simulink model "x_33_sim"  (R2016b)
settings: Solver=VariableStepAuto  StartTime=0.0  StopTime=0.001  RelTol=1e-3
settings Model: Creator=djh  LastModifiedBy=djh

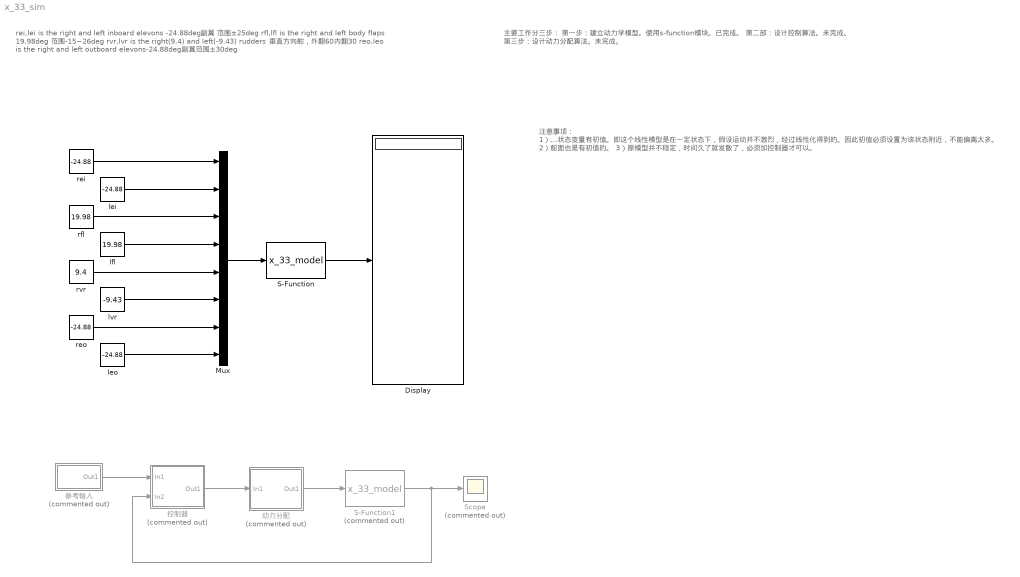
== system x_33_sim ==
  note: rei,lei is the right and left inboard elevons -24.88deg副翼 范围±25deg
      | rfl,lfl is the right and left body flaps 19.98deg 范围-15~26deg
      | rvr,lvr is the right(9.4) and left(-9.43) rudders 垂直方向舵，外翻60内翻30
      | reo,leo is the right and left outboard elevons-24.88deg副翼范围±30deg
  note: 主要工作分三步：
      | 第一步：建立动力学模型。使用s-function模块。已完成。
      | 第二部：设计控制算法。未完成。
      | 第三步：设计动力分配算法。未完成。
  note: 注意事项：
      | 1）状态变量有初值。即这个线性模型是在一定状态下，假设运动并不激烈，经过线性化得到的。因此初值必须设置为该状态附近，不能偏离太多。
      | 2）舵面也是有初值的。
      | 3）原模型并不稳定，时间久了就发散了，必须加控制器才可以。
  Display : Display
      settings: Decimation=17
  Mux : Mux  Inputs=8
  S-Function : S-Function  FunctionName=x_33_model  SFunctionDeploymentMode=off  EnableBusSupport=off
  S-Function1 : S-Function  Commented=on  FunctionName=x_33_model  SFunctionDeploymentMode=off  EnableBusSupport=off
  Scope : Scope  Commented=on
  lei : Constant  Value=-24.88
  leo : Constant  Value=-24.88
  lfl : Constant  Value=19.98
  lvr : Constant  Value=-9.43
  rei : Constant  Value=-24.88
  reo : Constant  Value=-24.88
  rfl : Constant  Value=19.98
  rvr : Constant  Value=9.4
  动力分配 : Subsystem  Commented=on
  参考输入 : Subsystem  Commented=on
  控制器 : Subsystem  Commented=on
  wires:
  S-Function/1 -> Display/1
  Mux/1 -> S-Function/1
  rei/1 -> Mux/1
  lei/1 -> Mux/2
  rfl/1 -> Mux/3
  lfl/1 -> Mux/4
  rvr/1 -> Mux/5
  lvr/1 -> Mux/6
  reo/1 -> Mux/7
  leo/1 -> Mux/8
  动力分配/1(Out1) -> S-Function1/1
  控制器/1(Out1) -> 动力分配/1(In1)
  参考输入/1(Out1) -> 控制器/1(In1)
  S-Function1/1 -> Scope/1, 控制器/2(In2)

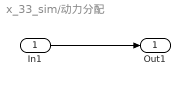
== system x_33_sim/动力分配 ==
  In1 : Inport
  Out1 : Outport
  wires:
  In1/1 -> Out1/1

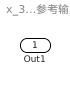
== system x_33_sim/参考输入 ==
  Out1 : Outport
  wires:
  ? -> Out1/1

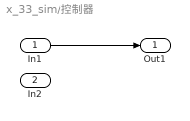
== system x_33_sim/控制器 ==
  In1 : Inport
  In2 : Inport  Port=2
  Out1 : Outport
  wires:
  In1/1 -> Out1/1
